simulink model "b6_pfc_rl"  (R2021b)
settings: Solver=FixedStepAuto  StartTime=0.0  StopTime=120.0  FixedStep=0.05  RelTol=1e-3
PreLoadFcn:
  | % Simulation parameters
  | %load exampleMap
  | 
  | % Lidar parameters
  | sensorOffset = [0,0];
  | scanAngles = linspace(-pi/2,pi/2,9)';
  | maxRange = 5;
InitFcn:
  | sampleTime = 0.05;
  | nMedianSize=3;
  | 
  | % Robot parameters
  | wheelRadius = 0.0335;
  | robotRadius = 0.116;
  | 
  | % Lidar parameters
  | sensorOffset = [0,0];
  | scanAngles = linspace(-pi/2,pi/2,9)';
  | maxRange = 5;
  | 
  | %%%%%%
  | ks=1;
  | c_ks=-1;
  | 
  | 
  | 
  | 
  | 
  | 
  | % Lidar parameters
  | sensorOffset = [0,0];
  | scanAngles = linspace(-pi/3,pi/3,20)';%y = linspace(x1,x2,n) 生成 n 个点。这些点的间距为 (x2-x1)/(n-1)。
  | maxRange = 0.4;
  | 
  | %%%%%%
  | ks=1;
  | 
  | 
  | 
  | 
  | 
  | A=0.3;
  | C=1.7;
  | B=(A+C)/2;
  | 
  | wp1=[A,A; B,A;  C,A; C,B;C,C; B,C; A,C;A,B];
  | bainjie2=[-0.5,-0.5;2.5,-0.5;-0.5,2.5;2.5,2.5;]
  | WAY_P=[wp1;wp1;wp1;wp1];
  | Target=[wp1;bainjie2];
  | 
  | %%%%%%%%%%%%%%%%%%%%%%%%%%%%%%%%%%%%%%%
  | Target_robot_4=[A  A]
  | Target_robot_5=[B  A]
  | Target_robot_6=[C  A]
  | 
  | Target_robot_1=[C  C]
  | Target_robot_2=[B  C]
  | Target_robot_3=[A  C]
  | 
  | 
  | %%%%%%%%%%%%%%%%%%%%%%%%%%%%%%%%%%%%
  | 
  | 
  | 
  | 
  | 
  | % paremeters of pure persuit
  | desired_v_robot_1=0.2
  | desired_w_robot_1=4
  | desired_lookahead_robot_1=0.2
  | 
  | % paremeters of recovery
  | recovery_w=0.5
  | 
  | 
  | 
  | 
  | 
  | %初始位置
  | x_1_0=1;
  | y_1_0=0;
  | yaw_1_0=0.0;
  | 
  | x_2_0=0.6;
  | y_2_0=0;
  | yaw_2_0=0;
  | 
  | x_3_0=0.3;
  | y_3_0=0;
  | yaw_3_0=0;
  | 
  | x_4_0=0;
  | y_4_0=0;
  | yaw_4_0=0;
  | 
  | x_5_0=-0.3;
  | y_5_0=0;
  | yaw_5_0=0;
  | 
  | x_6_0=-0.6;
  | y_6_0=0;
  | yaw_6_0=0;
  | 
  | init_pose_1=[x_1_0   y_1_0  yaw_1_0]';
  | init_pose_2=[x_2_0   y_2_0  yaw_2_0]';
  | init_pose_3=[x_3_0   y_3_0  yaw_3_0]';
  | init_pose_4=[x_4_0   y_4_0  yaw_4_0]';
  | 
  | init_pose_5=[x_5_0   y_5_0  yaw_5_0]';
  | init_pose_6=[x_6_0   y_6_0  yaw_6_0]';
undefined symbols (not defined in the file or in its folder): Angular, DiscIntNeverNeededParam, Linear, Pose, Twist
libraries: robotlib x42, dspstat3 x18, mobileRoboticsLib x13, robotmobilelib x6, simulink x2, robotalgslib x1
(part 1 of 3)
settings Model: Creator=scastro  LastModifiedBy=FCS
settings SolverCC: AlgebraicLoopSolver=TrustRegion
settings DataIOCC: ReturnWorkspaceOutputs=off
settings OptimizationCC: DefaultParameterBehavior=Inlined  EnhancedBackFolding=on  PassReuseOutputArgsAs=Individual arguments  ZeroExternalMemoryAtStartup=off  ZeroInternalMemoryAtStartup=off  InitFltsAndDblsToZero=on  MaxStackSize=64  OptimizeBlockOrder=speed  DifferentSizesBufferReuse=on  OptimizationCustomize=off  EfficientTunableParamExpr=on
settings DebuggingCC: ParameterTunabilityLossMsg=error  PregeneratedLibrarySubsystemCodeDiagnostic=none  SFMachineParentedDataDiag=warning  ArithmeticOperatorsInVariantConditions=warning
settings HardwareCC: ProdBitPerPointer=32  ProdBitPerSizeT=32  ProdBitPerPtrDiffT=32  ProdLargestAtomicFloat=None  ProdIntDivRoundTo=Undefined  ProdEndianess=Unspecified  ProdWordSize=32  ProdLongLongMode=on  ProdHWDeviceType=Generic->Unspecified (assume 32-bit Generic)  TargetLongLongMode=on
settings SFSimCC: SimUseLocalCustomCode=off  MATLABDynamicMemAlloc=off  CustomCodeUndefinedFunction=UseInterfaceOnly  SimTargetLang=C++
settings RTWCC: Description=Embedded Coder  SystemTargetFile=ert.tlc  HardwareBoard=Robot Operating System (ROS)  TLCOptions="-aInlineSetEventsForThisBaseRateFcn=TLC_FALSE -aSuppressMultiTaskScheduler=TLC_FALSE  -aRateBasedStepFcn=0"  TemplateMakefile=ert_default_tmf  RTWUseLocalCustomCode=off  Toolchain=Catkin  TargetLang=C++  GenerateGPUCode=CUDA
settings CodeAppCC: ForceParamTrailComments=on  IgnoreCustomStorageClasses=off  OperatorAnnotations=on  SimulinkDataObjDesc=on  SFDataObjDesc=on  InsertBlockDesc=on
settings ERTTargetCC: TargetLangStandard=C++11 (ISO)  CodeInterfacePackaging=C++ class  InlinedParameterPlacement=NonHierarchical  RootIOFormat=Structure reference  ERTCustomFileTemplate=example_file_process.tlc

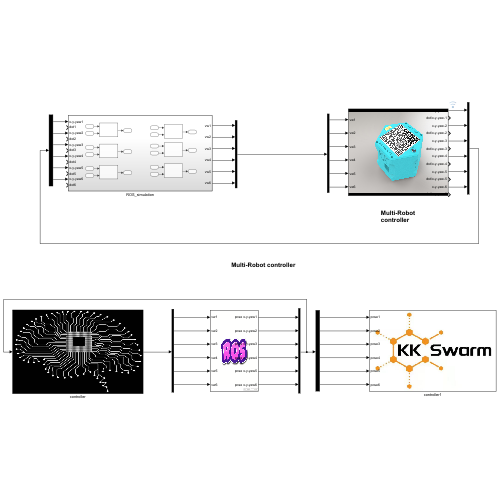
[thumbnail: Simulink's stored preview of the top-level diagram]
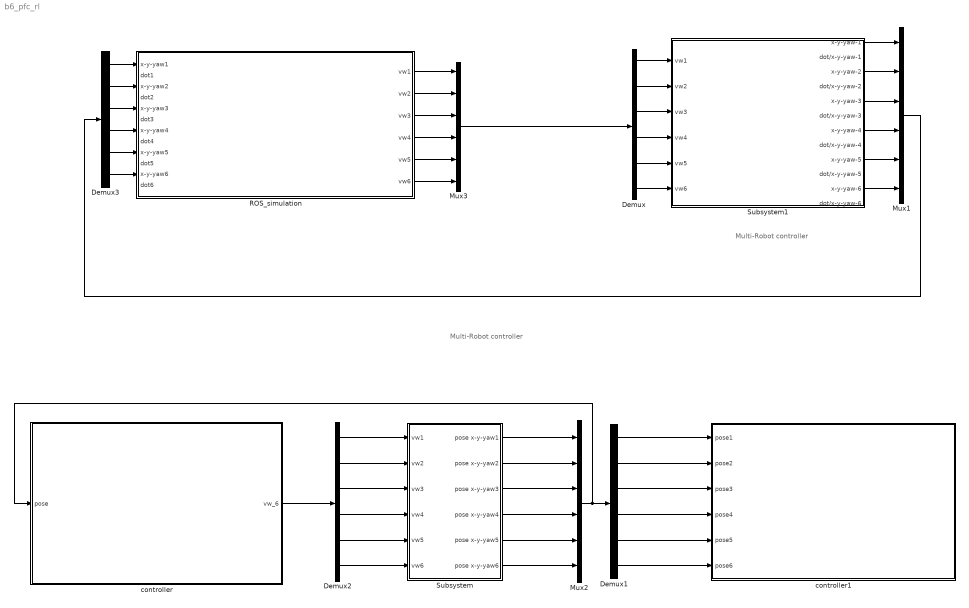
== system b6_pfc_rl ==
  note: Multi-Robot
      | controller
  note: Multi-Robot controller
  Demux{,1..3} (4 alike) : Demux  Outputs=6
  Mux1 : Mux  Inputs=6
  Mux2 : Mux  Inputs=6
  Mux3 : Mux  Inputs=6
  ROS_simulation : Subsystem
  Subsystem : Subsystem
      mask Display: image('$imagefile'); % 使用工具条上的 "编辑图像" 进行更改。
  Subsystem1 : Subsystem
      mask Display: image('$imagefile'); % 使用工具条上的 "编辑图像" 进行更改。
  controller : Subsystem
      mask Display: image('$imagefile'); % 使用工具条上的 "编辑图像" 进行更改。
  controller1 : Subsystem
      mask Display: image('$imagefile'); % 使用工具条上的 "编辑图像" 进行更改。
  wires:
  Demux/6 -> Subsystem1/6(vw6)
  ROS_simulation/3(vw3) -> Mux3/3
  Demux3/3 -> ROS_simulation/5(x-y-yaw3)
  Demux3/6 -> ROS_simulation/11(x-y-yaw6)
  Subsystem1/5(x-y-yaw-3) -> Mux1/3
  ROS_simulation/1(vw1) -> Mux3/1
  Mux3/1 -> Demux/1
  Demux/3 -> Subsystem1/3(vw3)
  Demux/4 -> Subsystem1/4(vw4)
  Demux3/4 -> ROS_simulation/7(x-y-yaw4)
  Mux1/1 -> Demux3/1
  Subsystem1/7(x-y-yaw-4) -> Mux1/4
  Demux3/2 -> ROS_simulation/3(x-y-yaw2)
  ROS_simulation/4(vw4) -> Mux3/4
  ROS_simulation/2(vw2) -> Mux3/2
  Demux/5 -> Subsystem1/5(vw5)
  Subsystem1/1(x-y-yaw-1) -> Mux1/1
  Demux/1 -> Subsystem1/1(vw1)
  ROS_simulation/6(vw6) -> Mux3/6
  ROS_simulation/5(vw5) -> Mux3/5
  Subsystem1/9(x-y-yaw-5) -> Mux1/5
  Demux/2 -> Subsystem1/2(vw2)
  Demux3/1 -> ROS_simulation/1(x-y-yaw1)
  Subsystem1/11(x-y-yaw-6) -> Mux1/6
  Demux3/5 -> ROS_simulation/9(x-y-yaw5)
  Subsystem1/3(x-y-yaw-2) -> Mux1/2
  Demux1/6 -> controller1/6(pose6)
  Subsystem/2(pose x-y-yaw2) -> Mux2/2
  Demux2/4 -> Subsystem/4(vw4)
  Demux1/5 -> controller1/5(pose5)
  Demux2/6 -> Subsystem/6(vw6)
  Mux2/1 -> controller/1(pose), Demux1/1
  Demux2/3 -> Subsystem/3(vw3)
  Demux1/4 -> controller1/4(pose4)
  Demux2/2 -> Subsystem/2(vw2)
  Demux2/5 -> Subsystem/5(vw5)
  Subsystem/4(pose x-y-yaw4) -> Mux2/4
  Demux1/3 -> controller1/3(pose3)
  Subsystem/6(pose x-y-yaw6) -> Mux2/6
  Demux1/1 -> controller1/1(pose1)
  Subsystem/1(pose x-y-yaw1) -> Mux2/1
  Subsystem/3(pose x-y-yaw3) -> Mux2/3
  Subsystem/5(pose x-y-yaw5) -> Mux2/5
  Demux1/2 -> controller1/2(pose2)
  Demux2/1 -> Subsystem/1(vw1)
  controller/1(vw_6) -> Demux2/1

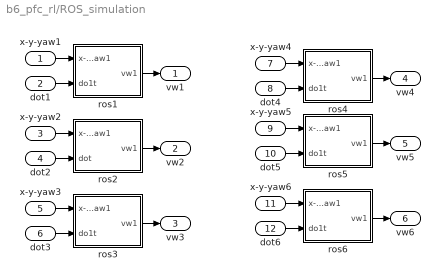
== system b6_pfc_rl/ROS_simulation ==
  x-y-yaw1 : Inport
  dot1 : Inport  Port=2
  x-y-yaw2 : Inport  Port=3
  dot2 : Inport  Port=4
  x-y-yaw3 : Inport  Port=5
  dot3 : Inport  Port=6
  x-y-yaw4 : Inport  Port=7
  dot4 : Inport  Port=8
  x-y-yaw5 : Inport  Port=9
  dot5 : Inport  Port=10
  x-y-yaw6 : Inport  Port=11
  dot6 : Inport  Port=12
  ros1 : Subsystem
  ros2 : Subsystem
  ros3 : Subsystem
  ros4 : Subsystem
  ros5 : Subsystem
  ros6 : Subsystem
  vw1 : Outport
  vw2 : Outport  Port=2
  vw3 : Outport  Port=3
  vw4 : Outport  Port=4
  vw5 : Outport  Port=5
  vw6 : Outport  Port=6
  wires:
  ros5/1(vw1) -> vw5/1
  ros2/1(vw1) -> vw2/1
  dot3/1 -> ros3/2(do1t)
  x-y-yaw5/1 -> ros5/1(x-y-yaw1)
  ros3/1(vw1) -> vw3/1
  dot2/1 -> ros2/2(dot)
  x-y-yaw2/1 -> ros2/1(x-y-yaw1)
  dot5/1 -> ros5/2(do1t)
  dot4/1 -> ros4/2(do1t)
  x-y-yaw4/1 -> ros4/1(x-y-yaw1)
  ros4/1(vw1) -> vw4/1
  x-y-yaw3/1 -> ros3/1(x-y-yaw1)
  dot6/1 -> ros6/2(do1t)
  x-y-yaw6/1 -> ros6/1(x-y-yaw1)
  dot1/1 -> ros1/2(do1t)
  ros6/1(vw1) -> vw6/1
  x-y-yaw1/1 -> ros1/1(x-y-yaw1)
  ros1/1(vw1) -> vw1/1

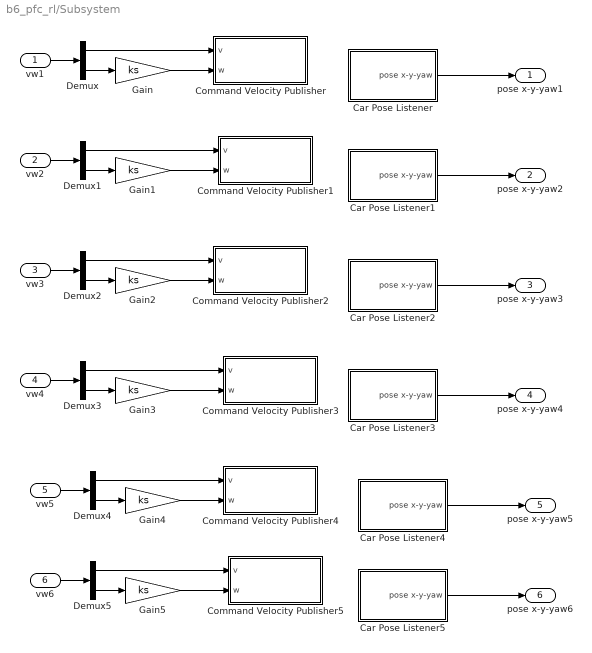
== system b6_pfc_rl/Subsystem ==
  vw1 : Inport
  vw2 : Inport  Port=2
  vw3 : Inport  Port=3
  vw4 : Inport  Port=4
  vw5 : Inport  Port=5
  vw6 : Inport  Port=6
  Car Pose Listener : Subsystem
  Car Pose Listener1 : Subsystem
  Car Pose Listener2 : Subsystem
  Car Pose Listener3 : Subsystem
  Car Pose Listener4 : Subsystem
  Car Pose Listener5 : Subsystem
  Command Velocity Publisher : Subsystem
  Command Velocity Publisher1 : Subsystem
  Command Velocity Publisher2 : Subsystem
  Command Velocity Publisher3 : Subsystem
  Command Velocity Publisher4 : Subsystem
  Command Velocity Publisher5 : Subsystem
  Demux{,1..5} (6 alike) : Demux  Outputs=2
  Gain{,1..5} (6 alike) : Gain  Gain=ks
  pose x-y-yaw1 : Outport
  pose x-y-yaw2 : Outport  Port=2
  pose x-y-yaw3 : Outport  Port=3
  pose x-y-yaw4 : Outport  Port=4
  pose x-y-yaw5 : Outport  Port=5
  pose x-y-yaw6 : Outport  Port=6
  wires:
  Gain/1 -> Command Velocity Publisher/2(w)
  Demux/2 -> Gain/1
  Car Pose Listener/1(pose x-y-yaw) -> pose x-y-yaw1/1
  Demux/1 -> Command Velocity Publisher/1(v)
  vw1/1 -> Demux/1
  Car Pose Listener1/1(pose x-y-yaw) -> pose x-y-yaw2/1
  Gain1/1 -> Command Velocity Publisher1/2(w)
  vw2/1 -> Demux1/1
  Demux1/2 -> Gain1/1
  Demux1/1 -> Command Velocity Publisher1/1(v)
  Car Pose Listener2/1(pose x-y-yaw) -> pose x-y-yaw3/1
  Gain2/1 -> Command Velocity Publisher2/2(w)
  vw3/1 -> Demux2/1
  Demux2/2 -> Gain2/1
  Demux2/1 -> Command Velocity Publisher2/1(v)
  Car Pose Listener3/1(pose x-y-yaw) -> pose x-y-yaw4/1
  Gain3/1 -> Command Velocity Publisher3/2(w)
  vw4/1 -> Demux3/1
  Demux3/2 -> Gain3/1
  Demux3/1 -> Command Velocity Publisher3/1(v)
  Car Pose Listener4/1(pose x-y-yaw) -> pose x-y-yaw5/1
  Gain4/1 -> Command Velocity Publisher4/2(w)
  vw5/1 -> Demux4/1
  Demux4/2 -> Gain4/1
  Car Pose Listener5/1(pose x-y-yaw) -> pose x-y-yaw6/1
  Gain5/1 -> Command Velocity Publisher5/2(w)
  vw6/1 -> Demux5/1
  Demux5/2 -> Gain5/1
  Demux5/1 -> Command Velocity Publisher5/1(v)
  Demux4/1 -> Command Velocity Publisher4/1(v)

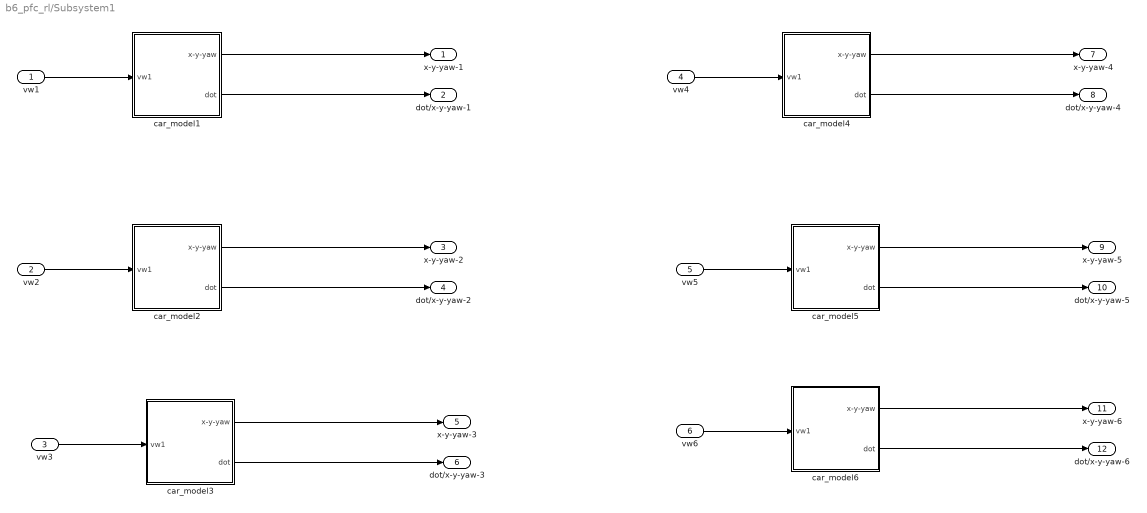
== system b6_pfc_rl/Subsystem1 ==
  vw1 : Inport
  vw2 : Inport  Port=2
  vw3 : Inport  Port=3
  vw4 : Inport  Port=4
  vw5 : Inport  Port=5
  vw6 : Inport  Port=6
  car_model1 : Subsystem
  car_model2 : Subsystem
  car_model3 : Subsystem
  car_model4 : Subsystem
  car_model5 : Subsystem
  car_model6 : Subsystem
  x-y-yaw-1 : Outport
  dot/x-y-yaw-1 : Outport  Port=2
  x-y-yaw-2 : Outport  Port=3
  dot/x-y-yaw-2 : Outport  Port=4
  x-y-yaw-3 : Outport  Port=5
  dot/x-y-yaw-3 : Outport  Port=6
  x-y-yaw-4 : Outport  Port=7
  dot/x-y-yaw-4 : Outport  Port=8
  x-y-yaw-5 : Outport  Port=9
  dot/x-y-yaw-5 : Outport  Port=10
  x-y-yaw-6 : Outport  Port=11
  dot/x-y-yaw-6 : Outport  Port=12
  wires:
  car_model1/1(x-y-yaw) -> x-y-yaw-1/1
  vw1/1 -> car_model1/1(vw1)
  car_model1/2(dot) -> dot/x-y-yaw-1/1
  car_model2/2(dot) -> dot/x-y-yaw-2/1
  vw2/1 -> car_model2/1(vw1)
  car_model2/1(x-y-yaw) -> x-y-yaw-2/1
  car_model3/1(x-y-yaw) -> x-y-yaw-3/1
  vw3/1 -> car_model3/1(vw1)
  car_model3/2(dot) -> dot/x-y-yaw-3/1
  car_model4/1(x-y-yaw) -> x-y-yaw-4/1
  vw4/1 -> car_model4/1(vw1)
  car_model4/2(dot) -> dot/x-y-yaw-4/1
  car_model5/1(x-y-yaw) -> x-y-yaw-5/1
  vw5/1 -> car_model5/1(vw1)
  car_model5/2(dot) -> dot/x-y-yaw-5/1
  car_model6/1(x-y-yaw) -> x-y-yaw-6/1
  vw6/1 -> car_model6/1(vw1)
  car_model6/2(dot) -> dot/x-y-yaw-6/1

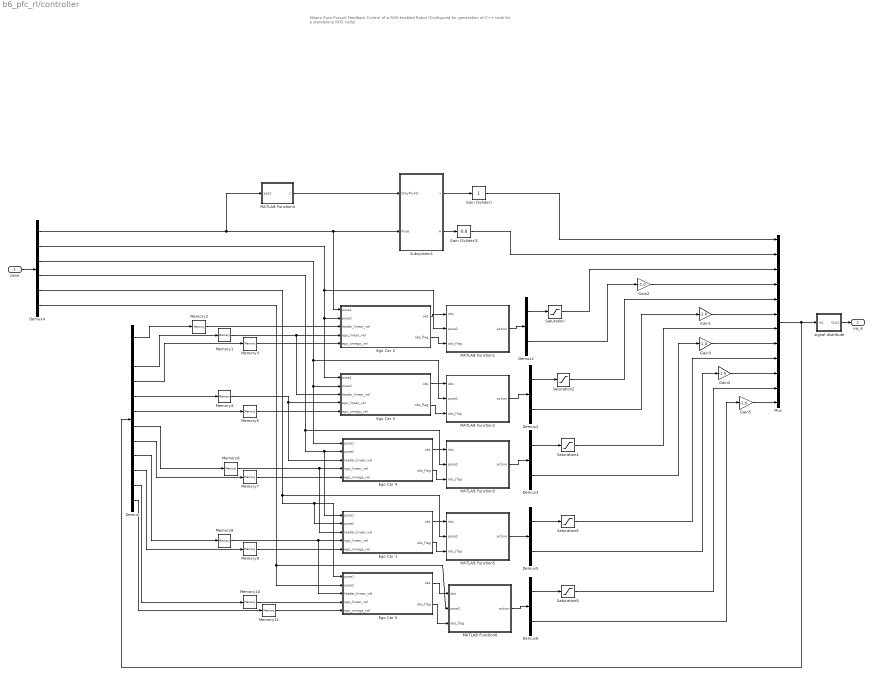
== system b6_pfc_rl/controller ==
  note: Misaro Pure Pursuit Feedback Control of a ROS-enabled Robot
      | (Configured for generation of C++ code for a standalone ROS node)
  pose : Inport
  Demux : Demux  Outputs=12
  Demux{1..3,5..6} (5 alike) : Demux  Outputs=2
  Demux4 : Demux  Outputs=6
  Ego Car 1 : Subsystem
  Ego Car 2 : Subsystem
  Ego Car 3 : Subsystem
  Ego Car 4 : Subsystem
  Ego Car 5 : Subsystem
  Gain (Svlider) : simulink/Math Operations/Slider Gain  gain=1  low=0.1  high=10
  Gain (Svlider)1 : simulink/Math Operations/Slider Gain  gain=0.8  low=0.1  high=3
  Gain{1..5} (5 alike) : Gain  Gain=-1.0
  MATLAB Function1 : MATLAB Function  TreatAsAtomicUnit=on
  MATLAB Function2 : MATLAB Function  TreatAsAtomicUnit=on
  MATLAB Function3 : MATLAB Function  TreatAsAtomicUnit=on
  MATLAB Function4 : MATLAB Function  TreatAsAtomicUnit=on
  MATLAB Function5 : MATLAB Function  TreatAsAtomicUnit=on
  MATLAB Function6 : MATLAB Function  TreatAsAtomicUnit=on
  Memory{1..2,4,6,8,10} (6 alike) : Memory  InitialCondition=0.2
  Memory{3,5,7,9,11} (5 alike) : Memory
  Mux : Mux  Inputs=12
  Saturation{,2,4,6,8} (5 alike) : Saturate  LowerLimit=0.1  OutDataTypeStr=double
  Subsystem1 : Subsystem
  signal distribute : Subsystem
  vw_6 : Outport
  wires:
  Demux4/1 -> MATLAB Function4/1(pos1), Ego Car 2/1(pose1), Subsystem1/2(Pose)
  Demux/1 -> Memory2/1
  Demux/3 -> Memory1/1
  Demux/4 -> Memory3/1
  Demux/5 -> Memory4/1
  Demux/6 -> Memory5/1
  Demux/7 -> Memory6/1
  Demux/8 -> Memory7/1
  Demux4/2 -> MATLAB Function1/2(pose2), Ego Car 3/1(pose1), Ego Car 2/2(pose2)
  Demux4/3 -> MATLAB Function2/2(pose2), Ego Car 4/1(pose1), Ego Car 3/2(pose2)
  Demux4/4 -> MATLAB Function3/2(pose2), Ego Car 1/1(pose1), Ego Car 4/2(pose2)
  Subsystem1/1(v) -> Gain (Svlider)/1
  Memory2/1 -> Ego Car 2/3(leader_linear_vel)
  Memory1/1 -> Ego Car 3/3(leader_linear_vel), Ego Car 2/4(ego_linear_vel)
  Memory3/1 -> Ego Car 2/5(ego_omega_vel)
  Demux1/1 -> Saturation/1
  Saturation/1 -> Mux/3
  Subsystem1/2(w) -> Gain (Svlider)1/1
  Demux1/2 -> Gain2/1
  Memory4/1 -> Ego Car 4/3(leader_linear_vel), Ego Car 3/4(ego_linear_vel)
  Memory5/1 -> Ego Car 3/5(ego_omega_vel)
  Demux2/1 -> Saturation2/1
  Saturation2/1 -> Mux/5
  Demux2/2 -> Gain1/1
  Gain1/1 -> Mux/6
  Memory6/1 -> Ego Car 1/3(leader_linear_vel), Ego Car 4/4(ego_linear_vel)
  Memory7/1 -> Ego Car 4/5(ego_omega_vel)
  Demux3/1 -> Saturation4/1
  Saturation4/1 -> Mux/7
  Demux3/2 -> Gain3/1
  Gain3/1 -> Mux/8
  pose/1 -> Demux4/1
  Mux/1 -> Demux/1, signal distribute/1(In1)
  signal distribute/1(Out1) -> vw_6/1
  MATLAB Function4/1(z) -> Subsystem1/1(WayPoints)
  Gain (Svlider)/1 -> Mux/1
  Gain2/1 -> Mux/4
  Gain (Svlider)1/1 -> Mux/2
  Ego Car 3/1(obs) -> MATLAB Function2/1(obs)
  Ego Car 3/2(obs_flag) -> MATLAB Function2/3(obs_flag)
  MATLAB Function2/1(action) -> Demux2/1
  Ego Car 4/2(obs_flag) -> MATLAB Function3/3(obs_flag)
  Ego Car 4/1(obs) -> MATLAB Function3/1(obs)
  MATLAB Function3/1(action) -> Demux3/1
  MATLAB Function1/1(action) -> Demux1/1
  Ego Car 2/2(obs_flag) -> MATLAB Function1/3(obs_flag)
  Ego Car 2/1(obs) -> MATLAB Function1/1(obs)
  Demux/9 -> Memory8/1
  Demux/10 -> Memory9/1
  Memory8/1 -> Ego Car 5/3(leader_linear_vel), Ego Car 1/4(ego_linear_vel)
  Memory9/1 -> Ego Car 1/5(ego_omega_vel)
  Demux4/5 -> MATLAB Function5/2(pose2), Ego Car 5/1(pose1), Ego Car 1/2(pose2)
  Ego Car 1/1(obs) -> MATLAB Function5/1(obs)
  Ego Car 1/2(obs_flag) -> MATLAB Function5/3(obs_flag)
  Demux5/1 -> Saturation6/1
  MATLAB Function5/1(action) -> Demux5/1
  Saturation6/1 -> Mux/9
  Gain4/1 -> Mux/10
  Demux5/2 -> Gain4/1
  Demux/11 -> Memory10/1
  Memory10/1 -> Ego Car 5/4(ego_linear_vel)
  Demux/12 -> Memory11/1
  Memory11/1 -> Ego Car 5/5(ego_omega_vel)
  Demux4/6 -> MATLAB Function6/2(pose2), Ego Car 5/2(pose2)
  Ego Car 5/1(obs) -> MATLAB Function6/1(obs)
  Ego Car 5/2(obs_flag) -> MATLAB Function6/3(obs_flag)
  Demux6/1 -> Saturation8/1
  MATLAB Function6/1(action) -> Demux6/1
  Saturation8/1 -> Mux/11
  Gain5/1 -> Mux/12
  Demux6/2 -> Gain5/1

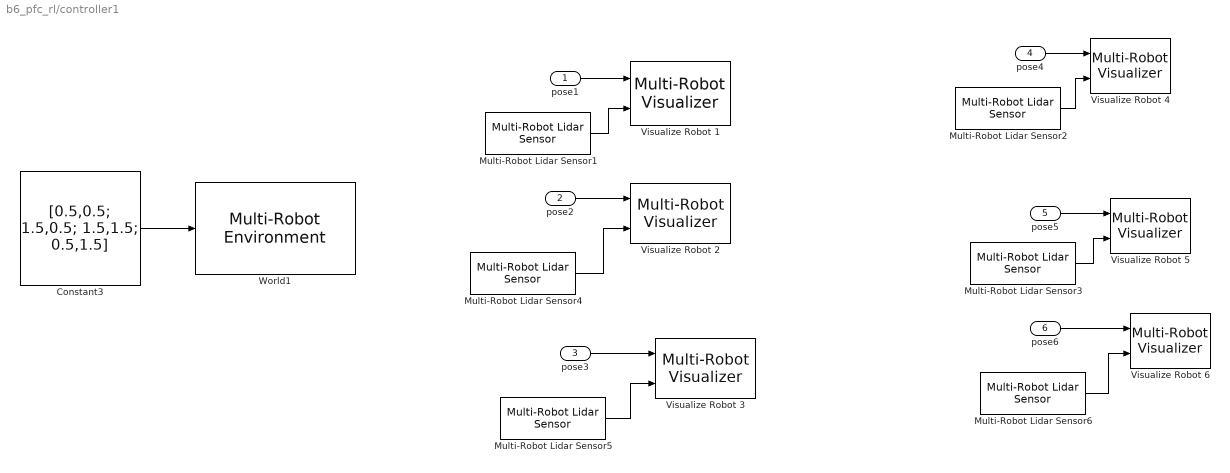
== system b6_pfc_rl/controller1 ==
  pose1 : Inport
  pose2 : Inport  Port=2
  pose3 : Inport  Port=3
  pose4 : Inport  Port=4
  pose5 : Inport  Port=5
  pose6 : Inport  Port=6
  Constant3 : Constant  Value="[0.5,0.5; 1.5,0.5;  1.5,1.5;  0.5,1.5]"
  Multi-Robot Lidar Sensor1 : mobileRoboticsLib/Environments/Multi-Robot Lidar Sensor  robotIdx=1  sensorOffset=sensorOffset  scanAngles=scanAngles  maxRange=maxRange
      settings: SourceProductName=Mobile Robotics Simulation Toolbox
  Multi-Robot Lidar Sensor2 : mobileRoboticsLib/Environments/Multi-Robot Lidar Sensor  robotIdx=4  sensorOffset=sensorOffset  scanAngles=scanAngles  maxRange=maxRange
      settings: SourceProductName=Mobile Robotics Simulation Toolbox
  Multi-Robot Lidar Sensor3 : mobileRoboticsLib/Environments/Multi-Robot Lidar Sensor  robotIdx=5  sensorOffset=sensorOffset  scanAngles=scanAngles  maxRange=maxRange
      settings: SourceProductName=Mobile Robotics Simulation Toolbox
  Multi-Robot Lidar Sensor4 : mobileRoboticsLib/Environments/Multi-Robot Lidar Sensor  robotIdx=2  sensorOffset=sensorOffset  scanAngles=scanAngles  maxRange=maxRange
      settings: SourceProductName=Mobile Robotics Simulation Toolbox
  Multi-Robot Lidar Sensor5 : mobileRoboticsLib/Environments/Multi-Robot Lidar Sensor  robotIdx=3  sensorOffset=sensorOffset  scanAngles=scanAngles  maxRange=maxRange
      settings: SourceProductName=Mobile Robotics Simulation Toolbox
  Multi-Robot Lidar Sensor6 : mobileRoboticsLib/Environments/Multi-Robot Lidar Sensor  robotIdx=6  sensorOffset=sensorOffset  scanAngles=scanAngles  maxRange=maxRange
      settings: SourceProductName=Mobile Robotics Simulation Toolbox
  Visualize Robot 1 : mobileRoboticsLib/Environments/Multi-Robot Visualizer  idx=1  radius=robotRadius  robotColor=[0 0 1]  showTraj=off  hasLidar=on  sensorOffset=sensorOffset  scanAngles=scanAngles  maxNumScans=0  hasObjDetector=off  objDetectorOffset=[0,0]  objDetectorAngle=0  objDetectorFOV=pi/2  objDetectorMaxRange=5  hasRobotDetector=off  robotDetectorOffset=[0,0]  robotDetectorAngle=0  robotDetectorFOV=pi/3  robotDetectorMaxRange=5  robotDetectorNumDetections=0
      settings: SourceProductName=Mobile Robotics Simulation Toolbox
  Visualize Robot 2 : mobileRoboticsLib/Environments/Multi-Robot Visualizer  idx=2  radius=robotRadius  robotColor=[0 1 0]  showTraj=on  hasLidar=on  sensorOffset=sensorOffset  scanAngles=scanAngles  maxNumScans=0  hasObjDetector=off  objDetectorOffset=[0,0]  objDetectorAngle=0  objDetectorFOV=pi/2  objDetectorMaxRange=5  hasRobotDetector=off  robotDetectorOffset=[0,0]  robotDetectorAngle=0  robotDetectorFOV=pi/3  robotDetectorMaxRange=5  robotDetectorNumDetections=0
      settings: SourceProductName=Mobile Robotics Simulation Toolbox
  Visualize Robot 3 : mobileRoboticsLib/Environments/Multi-Robot Visualizer  idx=3  radius=robotRadius  robotColor=[0 1 0]  showTraj=off  hasLidar=on  sensorOffset=sensorOffset  scanAngles=scanAngles  maxNumScans=0  hasObjDetector=off  objDetectorOffset=[0,0]  objDetectorAngle=0  objDetectorFOV=pi/2  objDetectorMaxRange=5  hasRobotDetector=off  robotDetectorOffset=[0,0]  robotDetectorAngle=0  robotDetectorFOV=pi/3  robotDetectorMaxRange=5  robotDetectorNumDetections=0
      settings: SourceProductName=Mobile Robotics Simulation Toolbox
  Visualize Robot 4 : mobileRoboticsLib/Environments/Multi-Robot Visualizer  idx=4  radius=robotRadius  robotColor=[1 0 0]  showTraj=on  hasLidar=on  sensorOffset=sensorOffset  scanAngles=scanAngles  maxNumScans=0  hasObjDetector=off  objDetectorOffset=[0,0]  objDetectorAngle=0  objDetectorFOV=pi/2  objDetectorMaxRange=5  hasRobotDetector=off  robotDetectorOffset=[0,0]  robotDetectorAngle=0  robotDetectorFOV=pi/3  robotDetectorMaxRange=5  robotDetectorNumDetections=0
      settings: SourceProductName=Mobile Robotics Simulation Toolbox
  Visualize Robot 5 : mobileRoboticsLib/Environments/Multi-Robot Visualizer  idx=5  radius=robotRadius  robotColor=[1 0 1]  showTraj=off  hasLidar=on  sensorOffset=sensorOffset  scanAngles=scanAngles  maxNumScans=0  hasObjDetector=off  objDetectorOffset=[0,0]  objDetectorAngle=0  objDetectorFOV=pi/2  objDetectorMaxRange=5  hasRobotDetector=off  robotDetectorOffset=[0,0]  robotDetectorAngle=0  robotDetectorFOV=pi/3  robotDetectorMaxRange=5  robotDetectorNumDetections=0
      settings: SourceProductName=Mobile Robotics Simulation Toolbox
  Visualize Robot 6 : mobileRoboticsLib/Environments/Multi-Robot Visualizer  idx=6  radius=robotRadius  robotColor=[1 0 0]  showTraj=off  hasLidar=on  sensorOffset=sensorOffset  scanAngles=scanAngles  maxNumScans=0  hasObjDetector=off  objDetectorOffset=[0,0]  objDetectorAngle=0  objDetectorFOV=pi/2  objDetectorMaxRange=5  hasRobotDetector=off  robotDetectorOffset=[0,0]  robotDetectorAngle=0  robotDetectorFOV=pi/3  robotDetectorMaxRange=5  robotDetectorNumDetections=0
      settings: SourceProductName=Mobile Robotics Simulation Toolbox
  World1 : mobileRoboticsLib/Environments/Multi-Robot Environment  numRobots=6  showWaypoints=on  showObjects=off  objectColors=[1 0 0;0 1 0;0 0 1]  objectMarkers='s'  showRobotIds=on  plotSensorLines=on
      settings: SourceProductName=Mobile Robotics Simulation Toolbox
  wires:
  Multi-Robot Lidar Sensor5/1 -> Visualize Robot 3/2
  Multi-Robot Lidar Sensor4/1 -> Visualize Robot 2/2
  pose2/1 -> Visualize Robot 2/1
  Multi-Robot Lidar Sensor1/1 -> Visualize Robot 1/2
  Multi-Robot Lidar Sensor6/1 -> Visualize Robot 6/2
  Multi-Robot Lidar Sensor2/1 -> Visualize Robot 4/2
  pose6/1 -> Visualize Robot 6/1
  pose1/1 -> Visualize Robot 1/1
  pose4/1 -> Visualize Robot 4/1
  pose5/1 -> Visualize Robot 5/1
  Multi-Robot Lidar Sensor3/1 -> Visualize Robot 5/2
  pose3/1 -> Visualize Robot 3/1
  Constant3/1 -> World1/1

== system b6_pfc_rl/ROS_simulation/ros1 ==
  x-y-yaw1 : Inport
  do1t : Inport  Port=2
  " [x y theta]" : Demux  Outputs=3
  " [x y theta]1" : Demux  Outputs=3
  Blank Message : robotlib/Blank Message  messageClass=Message  entityType=nav_msgs/Odometry  messageType=nav_msgs/Odometry  SampleTime=inf  legacyBusStruct=off
  Bus Assignment1 : BusAssignment  DialogController=Simulink.DDGSource_BusAssignment  AssignedSignals=Pose.Pose.Position.X,Pose.Pose.Position.Y,Pose.Pose.Orientation.Z,Pose.Pose.Orientation.W,Twist.Twist.Linear.X,Twist.Twist.Linear.Y,Twist.Twist.Angular.Z
  MATLAB Function : MATLAB Function  TreatAsAtomicUnit=on
  MATLAB Function3 : MATLAB Function  TreatAsAtomicUnit=on
  Mux6 : Mux  Inputs=2
  Publish2 : robotlib/Publish  topicSource=Specify your own  topic=/robot_1/pose  messageType=nav_msgs/Odometry  legacyBusStruct=off  messageQueueLength=105
  Subscribe1 : robotlib/Subscribe  topicSource=Specify your own  topic=/robot_1/cmd_vel  messageType=geometry_msgs/Twist  SampleTime=-1  legacyBusStruct=off  messageQueueLength=51
  Terminator : Terminator
  Terminator1 : Terminator
  Zero-Order Hold : ZeroOrderHold  SampleTime=0.1
  Zero-Order Hold1 : ZeroOrderHold  SampleTime=0.1
  vw1 : Outport
  wires:
  " [x y theta]"/1 -> Bus Assignment1/2
  Blank Message/1 -> Bus Assignment1/1
  x-y-yaw1/1 -> Zero-Order Hold/1
  " [x y theta]"/2 -> Bus Assignment1/3
  " [x y theta]1"/2 -> Bus Assignment1/7
  " [x y theta]"/3 -> MATLAB Function/1(yaw)
  " [x y theta]1"/3 -> Bus Assignment1/8
  MATLAB Function/4(w) -> Bus Assignment1/5
  MATLAB Function/3(z) -> Bus Assignment1/4
  " [x y theta]1"/1 -> Bus Assignment1/6
  Bus Assignment1/1 -> Publish2/1
  do1t/1 -> Zero-Order Hold1/1
  MATLAB Function/1(x) -> Terminator/1
  MATLAB Function/2(y) -> Terminator1/1
  Zero-Order Hold/1 -> " [x y theta]"/1
  Zero-Order Hold1/1 -> " [x y theta]1"/1
  Mux6/1 -> vw1/1
  MATLAB Function3/2(wref) -> Mux6/2
  MATLAB Function3/1(vref) -> Mux6/1
  Subscribe1/1 -> MATLAB Function3/1(IsNew)
  Subscribe1/2 -> MATLAB Function3/2(cmdMsg)

== system b6_pfc_rl/ROS_simulation/ros2 ==
  x-y-yaw1 : Inport
  dot : Inport  Port=2
  " [x y theta]" : Demux  Outputs=3
  " [x y theta]1" : Demux  Outputs=3
  Blank Message : robotlib/Blank Message  messageClass=Message  entityType=nav_msgs/Odometry  messageType=nav_msgs/Odometry  SampleTime=inf  legacyBusStruct=off
  Bus Assignment1 : BusAssignment  DialogController=Simulink.DDGSource_BusAssignment  AssignedSignals=Pose.Pose.Position.X,Pose.Pose.Position.Y,Pose.Pose.Orientation.Z,Pose.Pose.Orientation.W,Twist.Twist.Linear.X,Twist.Twist.Linear.Y,Twist.Twist.Angular.Z
  MATLAB Function : MATLAB Function  TreatAsAtomicUnit=on
  MATLAB Function3 : MATLAB Function  TreatAsAtomicUnit=on
  Mux6 : Mux  Inputs=2
  Publish2 : robotlib/Publish  topicSource=Specify your own  topic=/robot_2/pose  messageType=nav_msgs/Odometry  legacyBusStruct=off  messageQueueLength=105
  Subscribe1 : robotlib/Subscribe  topicSource=Specify your own  topic=/robot_2/cmd_vel  messageType=geometry_msgs/Twist  SampleTime=-1  legacyBusStruct=off  messageQueueLength=51
  Terminator : Terminator
  Terminator1 : Terminator
  Zero-Order Hold : ZeroOrderHold  SampleTime=0.1
  Zero-Order Hold1 : ZeroOrderHold  SampleTime=0.1
  vw1 : Outport
  wires:
  " [x y theta]"/1 -> Bus Assignment1/2
  Blank Message/1 -> Bus Assignment1/1
  x-y-yaw1/1 -> Zero-Order Hold/1
  " [x y theta]"/2 -> Bus Assignment1/3
  " [x y theta]1"/2 -> Bus Assignment1/7
  " [x y theta]"/3 -> MATLAB Function/1(yaw)
  " [x y theta]1"/3 -> Bus Assignment1/8
  MATLAB Function/4(w) -> Bus Assignment1/5
  MATLAB Function/3(z) -> Bus Assignment1/4
  " [x y theta]1"/1 -> Bus Assignment1/6
  Bus Assignment1/1 -> Publish2/1
  dot/1 -> Zero-Order Hold1/1
  MATLAB Function/1(x) -> Terminator/1
  MATLAB Function/2(y) -> Terminator1/1
  Zero-Order Hold/1 -> " [x y theta]"/1
  Zero-Order Hold1/1 -> " [x y theta]1"/1
  MATLAB Function3/1(vref) -> Mux6/1
  MATLAB Function3/2(wref) -> Mux6/2
  Subscribe1/1 -> MATLAB Function3/1(IsNew)
  Subscribe1/2 -> MATLAB Function3/2(cmdMsg)
  Mux6/1 -> vw1/1

== system b6_pfc_rl/ROS_simulation/ros3 ==
  x-y-yaw1 : Inport
  do1t : Inport  Port=2
  " [x y theta]" : Demux  Outputs=3
  " [x y theta]1" : Demux  Outputs=3
  Blank Message : robotlib/Blank Message  messageClass=Message  entityType=nav_msgs/Odometry  messageType=nav_msgs/Odometry  SampleTime=inf  legacyBusStruct=off
  Bus Assignment1 : BusAssignment  DialogController=Simulink.DDGSource_BusAssignment  AssignedSignals=Pose.Pose.Position.X,Pose.Pose.Position.Y,Pose.Pose.Orientation.Z,Pose.Pose.Orientation.W,Twist.Twist.Linear.X,Twist.Twist.Linear.Y,Twist.Twist.Angular.Z
  MATLAB Function : MATLAB Function  TreatAsAtomicUnit=on
  MATLAB Function3 : MATLAB Function  TreatAsAtomicUnit=on
  Mux6 : Mux  Inputs=2
  Publish2 : robotlib/Publish  topicSource=Specify your own  topic=/robot_3/pose  messageType=nav_msgs/Odometry  legacyBusStruct=off  messageQueueLength=105
  Subscribe1 : robotlib/Subscribe  topicSource=Specify your own  topic=/robot_3/cmd_vel  messageType=geometry_msgs/Twist  SampleTime=-1  legacyBusStruct=off  messageQueueLength=51
  Terminator : Terminator
  Terminator1 : Terminator
  Zero-Order Hold : ZeroOrderHold  SampleTime=0.1
  Zero-Order Hold1 : ZeroOrderHold  SampleTime=0.1
  vw1 : Outport
  wires:
  " [x y theta]"/1 -> Bus Assignment1/2
  Blank Message/1 -> Bus Assignment1/1
  x-y-yaw1/1 -> Zero-Order Hold/1
  " [x y theta]"/2 -> Bus Assignment1/3
  " [x y theta]1"/2 -> Bus Assignment1/7
  " [x y theta]"/3 -> MATLAB Function/1(yaw)
  " [x y theta]1"/3 -> Bus Assignment1/8
  MATLAB Function/4(w) -> Bus Assignment1/5
  MATLAB Function/3(z) -> Bus Assignment1/4
  " [x y theta]1"/1 -> Bus Assignment1/6
  Bus Assignment1/1 -> Publish2/1
  do1t/1 -> Zero-Order Hold1/1
  MATLAB Function/1(x) -> Terminator/1
  MATLAB Function/2(y) -> Terminator1/1
  Zero-Order Hold/1 -> " [x y theta]"/1
  Zero-Order Hold1/1 -> " [x y theta]1"/1
  MATLAB Function3/1(vref) -> Mux6/1
  MATLAB Function3/2(wref) -> Mux6/2
  Subscribe1/1 -> MATLAB Function3/1(IsNew)
  Subscribe1/2 -> MATLAB Function3/2(cmdMsg)
  Mux6/1 -> vw1/1

== system b6_pfc_rl/ROS_simulation/ros4 ==
  x-y-yaw1 : Inport
  do1t : Inport  Port=2
  " [x y theta]" : Demux  Outputs=3
  " [x y theta]1" : Demux  Outputs=3
  Blank Message : robotlib/Blank Message  messageClass=Message  entityType=nav_msgs/Odometry  messageType=nav_msgs/Odometry  SampleTime=inf  legacyBusStruct=off
  Bus Assignment1 : BusAssignment  DialogController=Simulink.DDGSource_BusAssignment  AssignedSignals=Pose.Pose.Position.X,Pose.Pose.Position.Y,Pose.Pose.Orientation.Z,Pose.Pose.Orientation.W,Twist.Twist.Linear.X,Twist.Twist.Linear.Y,Twist.Twist.Angular.Z
  MATLAB Function : MATLAB Function  TreatAsAtomicUnit=on
  MATLAB Function3 : MATLAB Function  TreatAsAtomicUnit=on
  Mux6 : Mux  Inputs=2
  Publish2 : robotlib/Publish  topicSource=Specify your own  topic=/robot_4/pose  messageType=nav_msgs/Odometry  legacyBusStruct=off  messageQueueLength=105
  Subscribe1 : robotlib/Subscribe  topicSource=Specify your own  topic=/robot_4/cmd_vel  messageType=geometry_msgs/Twist  SampleTime=-1  legacyBusStruct=off  messageQueueLength=51
  Terminator : Terminator
  Terminator1 : Terminator
  Zero-Order Hold : ZeroOrderHold  SampleTime=0.1
  Zero-Order Hold1 : ZeroOrderHold  SampleTime=0.1
  vw1 : Outport
  wires:
  " [x y theta]"/1 -> Bus Assignment1/2
  Blank Message/1 -> Bus Assignment1/1
  x-y-yaw1/1 -> Zero-Order Hold/1
  " [x y theta]"/2 -> Bus Assignment1/3
  " [x y theta]1"/2 -> Bus Assignment1/7
  " [x y theta]"/3 -> MATLAB Function/1(yaw)
  " [x y theta]1"/3 -> Bus Assignment1/8
  MATLAB Function/4(w) -> Bus Assignment1/5
  MATLAB Function/3(z) -> Bus Assignment1/4
  " [x y theta]1"/1 -> Bus Assignment1/6
  Bus Assignment1/1 -> Publish2/1
  do1t/1 -> Zero-Order Hold1/1
  MATLAB Function/1(x) -> Terminator/1
  MATLAB Function/2(y) -> Terminator1/1
  Zero-Order Hold/1 -> " [x y theta]"/1
  Zero-Order Hold1/1 -> " [x y theta]1"/1
  MATLAB Function3/1(vref) -> Mux6/1
  MATLAB Function3/2(wref) -> Mux6/2
  Subscribe1/1 -> MATLAB Function3/1(IsNew)
  Subscribe1/2 -> MATLAB Function3/2(cmdMsg)
  Mux6/1 -> vw1/1

== system b6_pfc_rl/ROS_simulation/ros5 ==
  x-y-yaw1 : Inport
  do1t : Inport  Port=2
  " [x y theta]" : Demux  Outputs=3
  " [x y theta]1" : Demux  Outputs=3
  Blank Message : robotlib/Blank Message  messageClass=Message  entityType=nav_msgs/Odometry  messageType=nav_msgs/Odometry  SampleTime=inf  legacyBusStruct=off
  Bus Assignment1 : BusAssignment  DialogController=Simulink.DDGSource_BusAssignment  AssignedSignals=Pose.Pose.Position.X,Pose.Pose.Position.Y,Pose.Pose.Orientation.Z,Pose.Pose.Orientation.W,Twist.Twist.Linear.X,Twist.Twist.Linear.Y,Twist.Twist.Angular.Z
  MATLAB Function : MATLAB Function  TreatAsAtomicUnit=on
  MATLAB Function3 : MATLAB Function  TreatAsAtomicUnit=on
  Mux6 : Mux  Inputs=2
  Publish2 : robotlib/Publish  topicSource=Specify your own  topic=/robot_5/pose  messageType=nav_msgs/Odometry  legacyBusStruct=off  messageQueueLength=105
  Subscribe1 : robotlib/Subscribe  topicSource=Specify your own  topic=/robot_5/cmd_vel  messageType=geometry_msgs/Twist  SampleTime=-1  legacyBusStruct=off  messageQueueLength=51
  Terminator : Terminator
  Terminator1 : Terminator
  Zero-Order Hold : ZeroOrderHold  SampleTime=0.1
  Zero-Order Hold1 : ZeroOrderHold  SampleTime=0.1
  vw1 : Outport
  wires:
  " [x y theta]"/1 -> Bus Assignment1/2
  Blank Message/1 -> Bus Assignment1/1
  x-y-yaw1/1 -> Zero-Order Hold/1
  " [x y theta]"/2 -> Bus Assignment1/3
  " [x y theta]1"/2 -> Bus Assignment1/7
  " [x y theta]"/3 -> MATLAB Function/1(yaw)
  " [x y theta]1"/3 -> Bus Assignment1/8
  MATLAB Function/4(w) -> Bus Assignment1/5
  MATLAB Function/3(z) -> Bus Assignment1/4
  " [x y theta]1"/1 -> Bus Assignment1/6
  Bus Assignment1/1 -> Publish2/1
  do1t/1 -> Zero-Order Hold1/1
  MATLAB Function/1(x) -> Terminator/1
  MATLAB Function/2(y) -> Terminator1/1
  Zero-Order Hold/1 -> " [x y theta]"/1
  Zero-Order Hold1/1 -> " [x y theta]1"/1
  MATLAB Function3/1(vref) -> Mux6/1
  MATLAB Function3/2(wref) -> Mux6/2
  Subscribe1/1 -> MATLAB Function3/1(IsNew)
  Subscribe1/2 -> MATLAB Function3/2(cmdMsg)
  Mux6/1 -> vw1/1

== system b6_pfc_rl/ROS_simulation/ros6 ==
  x-y-yaw1 : Inport
  do1t : Inport  Port=2
  " [x y theta]" : Demux  Outputs=3
  " [x y theta]1" : Demux  Outputs=3
  Blank Message : robotlib/Blank Message  messageClass=Message  entityType=nav_msgs/Odometry  messageType=nav_msgs/Odometry  SampleTime=inf  legacyBusStruct=off
  Bus Assignment1 : BusAssignment  DialogController=Simulink.DDGSource_BusAssignment  AssignedSignals=Pose.Pose.Position.X,Pose.Pose.Position.Y,Pose.Pose.Orientation.Z,Pose.Pose.Orientation.W,Twist.Twist.Linear.X,Twist.Twist.Linear.Y,Twist.Twist.Angular.Z
  MATLAB Function : MATLAB Function  TreatAsAtomicUnit=on
  MATLAB Function3 : MATLAB Function  TreatAsAtomicUnit=on
  Mux6 : Mux  Inputs=2
  Publish2 : robotlib/Publish  topicSource=Specify your own  topic=/robot_6/pose  messageType=nav_msgs/Odometry  legacyBusStruct=off  messageQueueLength=105
  Subscribe1 : robotlib/Subscribe  topicSource=Specify your own  topic=/robot_6/cmd_vel  messageType=geometry_msgs/Twist  SampleTime=-1  legacyBusStruct=off  messageQueueLength=51
  Terminator : Terminator
  Terminator1 : Terminator
  Zero-Order Hold : ZeroOrderHold  SampleTime=0.1
  Zero-Order Hold1 : ZeroOrderHold  SampleTime=0.1
  vw1 : Outport
  wires:
  " [x y theta]"/1 -> Bus Assignment1/2
  Blank Message/1 -> Bus Assignment1/1
  x-y-yaw1/1 -> Zero-Order Hold/1
  " [x y theta]"/2 -> Bus Assignment1/3
  " [x y theta]1"/2 -> Bus Assignment1/7
  " [x y theta]"/3 -> MATLAB Function/1(yaw)
  " [x y theta]1"/3 -> Bus Assignment1/8
  MATLAB Function/4(w) -> Bus Assignment1/5
  MATLAB Function/3(z) -> Bus Assignment1/4
  " [x y theta]1"/1 -> Bus Assignment1/6
  Bus Assignment1/1 -> Publish2/1
  do1t/1 -> Zero-Order Hold1/1
  MATLAB Function/1(x) -> Terminator/1
  MATLAB Function/2(y) -> Terminator1/1
  MATLAB Function3/1(vref) -> Mux6/1
  MATLAB Function3/2(wref) -> Mux6/2
  Subscribe1/1 -> MATLAB Function3/1(IsNew)
  Subscribe1/2 -> MATLAB Function3/2(cmdMsg)
  Mux6/1 -> vw1/1
  Zero-Order Hold/1 -> " [x y theta]"/1
  Zero-Order Hold1/1 -> " [x y theta]1"/1

== system b6_pfc_rl/Subsystem/Car Pose Listener ==
  Subscribe : robotlib/Subscribe  topicSource=Specify your own  topic=/robot_1/pose  messageType=nav_msgs/Odometry  SampleTime=-1  legacyBusStruct=off  messageQueueLength=51
  Subscribe1 : robotlib/Subscribe  topicSource=Specify your own  topic=/robot_1/odometry  messageType=geometry_msgs/Twist  SampleTime=-1  legacyBusStruct=off  messageQueueLength=51
  Subsystem : Subsystem
  pose x-y-yaw : Outport
  wires:
  Subscribe/1 -> Subsystem/1(poseNew)  "IsNew"
  Subscribe/2 -> Subsystem/2(poseMsg)
  Subscribe1/1 -> Subsystem/3(VW_New)  "IsNew"
  Subscribe1/2 -> Subsystem/4(VW_Msg)
  Subsystem/1(pose) -> pose x-y-yaw/1

== system b6_pfc_rl/Subsystem/Car Pose Listener1 ==
  Subscribe : robotlib/Subscribe  topicSource=Specify your own  topic=/robot_2/pose  messageType=nav_msgs/Odometry  SampleTime=-1  legacyBusStruct=off  messageQueueLength=51
  Subscribe1 : robotlib/Subscribe  topicSource=Specify your own  topic=/robot_2/odometry  messageType=geometry_msgs/Twist  SampleTime=-1  legacyBusStruct=off  messageQueueLength=51
  Subsystem : Subsystem
  pose x-y-yaw : Outport
  wires:
  Subscribe/1 -> Subsystem/1(poseNew)  "IsNew"
  Subscribe/2 -> Subsystem/2(poseMsg)
  Subscribe1/2 -> Subsystem/4(VW_Msg)
  Subscribe1/1 -> Subsystem/3(VW_New)  "IsNew"
  Subsystem/1(pose) -> pose x-y-yaw/1

== system b6_pfc_rl/Subsystem/Car Pose Listener2 ==
  Subscribe : robotlib/Subscribe  topicSource=Specify your own  topic=/robot_3/pose  messageType=nav_msgs/Odometry  SampleTime=-1  legacyBusStruct=off  messageQueueLength=51
  Subscribe1 : robotlib/Subscribe  topicSource=Specify your own  topic=/robot_3/odometry  messageType=geometry_msgs/Twist  SampleTime=-1  legacyBusStruct=off  messageQueueLength=51
  Subsystem : Subsystem
  pose x-y-yaw : Outport
  wires:
  Subscribe/1 -> Subsystem/1(poseNew)  "IsNew"
  Subscribe/2 -> Subsystem/2(poseMsg)
  Subscribe1/1 -> Subsystem/3(VW_New)  "IsNew"
  Subscribe1/2 -> Subsystem/4(VW_Msg)
  Subsystem/1(pose) -> pose x-y-yaw/1

== system b6_pfc_rl/Subsystem/Car Pose Listener3 ==
  Subscribe : robotlib/Subscribe  topicSource=Specify your own  topic=/robot_4/pose  messageType=nav_msgs/Odometry  SampleTime=-1  legacyBusStruct=off  messageQueueLength=51
  Subscribe1 : robotlib/Subscribe  topicSource=Specify your own  topic=/robot_4/odometry  messageType=geometry_msgs/Twist  SampleTime=-1  legacyBusStruct=off  messageQueueLength=51
  Subsystem : Subsystem
  pose x-y-yaw : Outport
  wires:
  Subscribe/1 -> Subsystem/1(poseNew)  "IsNew"
  Subscribe/2 -> Subsystem/2(poseMsg)
  Subscribe1/1 -> Subsystem/3(VW_New)  "IsNew"
  Subscribe1/2 -> Subsystem/4(VW_Msg)
  Subsystem/1(pose) -> pose x-y-yaw/1

== system b6_pfc_rl/Subsystem/Car Pose Listener4 ==
  Subscribe : robotlib/Subscribe  topicSource=Specify your own  topic=/robot_5/pose  messageType=nav_msgs/Odometry  SampleTime=-1  legacyBusStruct=off  messageQueueLength=51
  Subscribe1 : robotlib/Subscribe  topicSource=Specify your own  topic=/robot_5/odometry  messageType=geometry_msgs/Twist  SampleTime=-1  legacyBusStruct=off  messageQueueLength=51
  Subsystem : Subsystem
  pose x-y-yaw : Outport
  wires:
  Subscribe/1 -> Subsystem/1(poseNew)  "IsNew"
  Subscribe/2 -> Subsystem/2(poseMsg)
  Subscribe1/1 -> Subsystem/3(VW_New)  "IsNew"
  Subscribe1/2 -> Subsystem/4(VW_Msg)
  Subsystem/1(pose) -> pose x-y-yaw/1

== system b6_pfc_rl/Subsystem/Car Pose Listener5 ==
  Subscribe : robotlib/Subscribe  topicSource=Specify your own  topic=/robot_6/pose  messageType=nav_msgs/Odometry  SampleTime=-1  legacyBusStruct=off  messageQueueLength=51
  Subscribe1 : robotlib/Subscribe  topicSource=Specify your own  topic=/robot_6/odometry  messageType=geometry_msgs/Twist  SampleTime=-1  legacyBusStruct=off  messageQueueLength=51
  Subsystem : Subsystem
  pose x-y-yaw : Outport
  wires:
  Subscribe/1 -> Subsystem/1(poseNew)  "IsNew"
  Subscribe/2 -> Subsystem/2(poseMsg)
  Subscribe1/1 -> Subsystem/3(VW_New)  "IsNew"
  Subscribe1/2 -> Subsystem/4(VW_Msg)
  Subsystem/1(pose) -> pose x-y-yaw/1

== system b6_pfc_rl/Subsystem/Command Velocity Publisher ==
  v : Inport
  w : Inport  Port=2
  Blank Message : robotlib/Blank Message  messageClass=Message  entityType=geometry_msgs/Twist  messageType=geometry_msgs/Twist  SampleTime=inf  legacyBusStruct=off
  Bus Assignment1 : BusAssignment  DialogController=Simulink.DDGSource_BusAssignment  AssignedSignals=Linear.X,Angular.Z
  Publish2 : robotlib/Publish  topicSource=Specify your own  topic=/robot_1/cmd_vel  messageType=geometry_msgs/Twist  legacyBusStruct=off  messageQueueLength=105
  wires:
  Bus Assignment1/1 -> Publish2/1
  Blank Message/1 -> Bus Assignment1/1
  v/1 -> Bus Assignment1/2
  w/1 -> Bus Assignment1/3

== system b6_pfc_rl/Subsystem/Command Velocity Publisher1 ==
  v : Inport
  w : Inport  Port=2
  Blank Message : robotlib/Blank Message  messageClass=Message  entityType=geometry_msgs/Twist  messageType=geometry_msgs/Twist  SampleTime=inf  legacyBusStruct=off
  Bus Assignment1 : BusAssignment  DialogController=Simulink.DDGSource_BusAssignment  AssignedSignals=Linear.X,Angular.Z
  Publish2 : robotlib/Publish  topicSource=Specify your own  topic=/robot_2/cmd_vel  messageType=geometry_msgs/Twist  legacyBusStruct=off  messageQueueLength=105
  wires:
  Bus Assignment1/1 -> Publish2/1
  Blank Message/1 -> Bus Assignment1/1
  v/1 -> Bus Assignment1/2
  w/1 -> Bus Assignment1/3

== system b6_pfc_rl/Subsystem/Command Velocity Publisher2 ==
  v : Inport
  w : Inport  Port=2
  Blank Message : robotlib/Blank Message  messageClass=Message  entityType=geometry_msgs/Twist  messageType=geometry_msgs/Twist  SampleTime=inf  legacyBusStruct=off
  Bus Assignment1 : BusAssignment  DialogController=Simulink.DDGSource_BusAssignment  AssignedSignals=Linear.X,Angular.Z
  Publish2 : robotlib/Publish  topicSource=Specify your own  topic=/robot_3/cmd_vel  messageType=geometry_msgs/Twist  legacyBusStruct=off  messageQueueLength=105
  wires:
  Bus Assignment1/1 -> Publish2/1
  Blank Message/1 -> Bus Assignment1/1
  v/1 -> Bus Assignment1/2
  w/1 -> Bus Assignment1/3

== system b6_pfc_rl/Subsystem/Command Velocity Publisher3 ==
  v : Inport
  w : Inport  Port=2
  Blank Message : robotlib/Blank Message  messageClass=Message  entityType=geometry_msgs/Twist  messageType=geometry_msgs/Twist  SampleTime=inf  legacyBusStruct=off
  Bus Assignment1 : BusAssignment  DialogController=Simulink.DDGSource_BusAssignment  AssignedSignals=Linear.X,Angular.Z
  Publish2 : robotlib/Publish  topicSource=Specify your own  topic=/robot_4/cmd_vel  messageType=geometry_msgs/Twist  legacyBusStruct=off  messageQueueLength=105
  wires:
  Bus Assignment1/1 -> Publish2/1
  Blank Message/1 -> Bus Assignment1/1
  v/1 -> Bus Assignment1/2
  w/1 -> Bus Assignment1/3

== system b6_pfc_rl/Subsystem/Command Velocity Publisher4 ==
  v : Inport
  w : Inport  Port=2
  Blank Message : robotlib/Blank Message  messageClass=Message  entityType=geometry_msgs/Twist  messageType=geometry_msgs/Twist  SampleTime=inf  legacyBusStruct=off
  Bus Assignment1 : BusAssignment  DialogController=Simulink.DDGSource_BusAssignment  AssignedSignals=Linear.X,Angular.Z
  Publish2 : robotlib/Publish  topicSource=Specify your own  topic=/robot_5/cmd_vel  messageType=geometry_msgs/Twist  legacyBusStruct=off  messageQueueLength=105
  wires:
  Bus Assignment1/1 -> Publish2/1
  Blank Message/1 -> Bus Assignment1/1
  v/1 -> Bus Assignment1/2
  w/1 -> Bus Assignment1/3

== system b6_pfc_rl/Subsystem/Command Velocity Publisher5 ==
  v : Inport
  w : Inport  Port=2
  Blank Message : robotlib/Blank Message  messageClass=Message  entityType=geometry_msgs/Twist  messageType=geometry_msgs/Twist  SampleTime=inf  legacyBusStruct=off
  Bus Assignment1 : BusAssignment  DialogController=Simulink.DDGSource_BusAssignment  AssignedSignals=Linear.X,Angular.Z
  Publish2 : robotlib/Publish  topicSource=Specify your own  topic=/robot_6/cmd_vel  messageType=geometry_msgs/Twist  legacyBusStruct=off  messageQueueLength=105
  wires:
  Bus Assignment1/1 -> Publish2/1
  Blank Message/1 -> Bus Assignment1/1
  v/1 -> Bus Assignment1/2
  w/1 -> Bus Assignment1/3

== system b6_pfc_rl/Subsystem1/car_model1 ==
  note: tr=0.6
      | 4T=0.6
      | 一阶系统的动态性能指标为：td=0.69T，tr=2.20T，ts=3T
  vw1 : Inport
  Demux : Demux  Outputs=2
  Differential Drive Kinematic Model1 : robotmobilelib/Differential Drive Kinematic Model  VehicleInputs=Vehicle Speed & Heading Angular Velocity  WheelRadius=wheelRadius  WheelSpeedRange=[-inf inf]  TrackWidth=robotRadius  InitialState=init_pose_1  SimulateUsing=Interpreted execution
      settings: SourceProductBaseCode=RO
  Simulink顺时针为正 小车逆时针为正 : Gain  Gain=ks
  Transfer Fcn : TransferFcn  Denominator=[0.15 1]
  Transfer Fcn1 : TransferFcn  Denominator=[0.16 1]
  x-y-yaw : Outport
  dot : Outport  Port=2
  wires:
  Simulink顺时针为正 小车逆时针为正/1 -> Transfer Fcn1/1
  Transfer Fcn/1 -> Differential Drive Kinematic Model1/1
  Demux/1 -> Transfer Fcn/1
  Transfer Fcn1/1 -> Differential Drive Kinematic Model1/2
  Demux/2 -> Simulink顺时针为正 小车逆时针为正/1
  vw1/1 -> Demux/1
  Differential Drive Kinematic Model1/1 -> x-y-yaw/1
  Differential Drive Kinematic Model1/2 -> dot/1

== system b6_pfc_rl/Subsystem1/car_model2 ==
  note: tr=0.6
      | 4T=0.6
      | 一阶系统的动态性能指标为：td=0.69T，tr=2.20T，ts=3T
  vw1 : Inport
  Demux : Demux  Outputs=2
  Differential Drive Kinematic Model1 : robotmobilelib/Differential Drive Kinematic Model  VehicleInputs=Vehicle Speed & Heading Angular Velocity  WheelRadius=wheelRadius  WheelSpeedRange=[-inf inf]  TrackWidth=robotRadius  InitialState=init_pose_2  SimulateUsing=Interpreted execution
      settings: SourceProductBaseCode=RO
  Simulink顺时针为正 小车逆时针为正 : Gain  Gain=ks
  Transfer Fcn : TransferFcn  Denominator=[0.15 1]
  Transfer Fcn1 : TransferFcn  Denominator=[0.16 1]
  x-y-yaw : Outport
  dot : Outport  Port=2
  wires:
  Simulink顺时针为正 小车逆时针为正/1 -> Transfer Fcn1/1
  Transfer Fcn/1 -> Differential Drive Kinematic Model1/1
  Demux/1 -> Transfer Fcn/1
  Transfer Fcn1/1 -> Differential Drive Kinematic Model1/2
  Demux/2 -> Simulink顺时针为正 小车逆时针为正/1
  vw1/1 -> Demux/1
  Differential Drive Kinematic Model1/1 -> x-y-yaw/1
  Differential Drive Kinematic Model1/2 -> dot/1

== system b6_pfc_rl/Subsystem1/car_model3 ==
  note: tr=0.6
      | 4T=0.6
      | 一阶系统的动态性能指标为：td=0.69T，tr=2.20T，ts=3T
  vw1 : Inport
  Demux : Demux  Outputs=2
  Differential Drive Kinematic Model1 : robotmobilelib/Differential Drive Kinematic Model  VehicleInputs=Vehicle Speed & Heading Angular Velocity  WheelRadius=wheelRadius  WheelSpeedRange=[-inf inf]  TrackWidth=robotRadius  InitialState=init_pose_3  SimulateUsing=Interpreted execution
      settings: SourceProductBaseCode=RO
  Simulink顺时针为正 小车逆时针为正 : Gain  Gain=ks
  Transfer Fcn : TransferFcn  Denominator=[0.15 1]
  Transfer Fcn1 : TransferFcn  Denominator=[0.16 1]
  x-y-yaw : Outport
  dot : Outport  Port=2
  wires:
  Simulink顺时针为正 小车逆时针为正/1 -> Transfer Fcn1/1
  Transfer Fcn/1 -> Differential Drive Kinematic Model1/1
  Demux/1 -> Transfer Fcn/1
  Transfer Fcn1/1 -> Differential Drive Kinematic Model1/2
  Demux/2 -> Simulink顺时针为正 小车逆时针为正/1
  vw1/1 -> Demux/1
  Differential Drive Kinematic Model1/1 -> x-y-yaw/1
  Differential Drive Kinematic Model1/2 -> dot/1

== system b6_pfc_rl/Subsystem1/car_model4 ==
  note: tr=0.6
      | 4T=0.6
      | 一阶系统的动态性能指标为：td=0.69T，tr=2.20T，ts=3T
  vw1 : Inport
  Demux : Demux  Outputs=2
  Differential Drive Kinematic Model1 : robotmobilelib/Differential Drive Kinematic Model  VehicleInputs=Vehicle Speed & Heading Angular Velocity  WheelRadius=wheelRadius  WheelSpeedRange=[-inf inf]  TrackWidth=robotRadius  InitialState=init_pose_4  SimulateUsing=Interpreted execution
      settings: SourceProductBaseCode=RO
  Simulink顺时针为正 小车逆时针为正 : Gain  Gain=ks
  Transfer Fcn : TransferFcn  Denominator=[0.15 1]
  Transfer Fcn1 : TransferFcn  Denominator=[0.16 1]
  x-y-yaw : Outport
  dot : Outport  Port=2
  wires:
  Simulink顺时针为正 小车逆时针为正/1 -> Transfer Fcn1/1
  Transfer Fcn/1 -> Differential Drive Kinematic Model1/1
  Demux/1 -> Transfer Fcn/1
  Transfer Fcn1/1 -> Differential Drive Kinematic Model1/2
  Demux/2 -> Simulink顺时针为正 小车逆时针为正/1
  vw1/1 -> Demux/1
  Differential Drive Kinematic Model1/1 -> x-y-yaw/1
  Differential Drive Kinematic Model1/2 -> dot/1

== system b6_pfc_rl/Subsystem1/car_model5 ==
  note: tr=0.6
      | 4T=0.6
      | 一阶系统的动态性能指标为：td=0.69T，tr=2.20T，ts=3T
  vw1 : Inport
  Demux : Demux  Outputs=2
  Differential Drive Kinematic Model1 : robotmobilelib/Differential Drive Kinematic Model  VehicleInputs=Vehicle Speed & Heading Angular Velocity  WheelRadius=wheelRadius  WheelSpeedRange=[-inf inf]  TrackWidth=robotRadius  InitialState=init_pose_5  SimulateUsing=Interpreted execution
      settings: SourceProductBaseCode=RO
  Simulink顺时针为正 小车逆时针为正 : Gain  Gain=ks
  Transfer Fcn : TransferFcn  Denominator=[0.15 1]
  Transfer Fcn1 : TransferFcn  Denominator=[0.16 1]
  x-y-yaw : Outport
  dot : Outport  Port=2
  wires:
  Simulink顺时针为正 小车逆时针为正/1 -> Transfer Fcn1/1
  Transfer Fcn/1 -> Differential Drive Kinematic Model1/1
  Demux/1 -> Transfer Fcn/1
  Transfer Fcn1/1 -> Differential Drive Kinematic Model1/2
  Demux/2 -> Simulink顺时针为正 小车逆时针为正/1
  vw1/1 -> Demux/1
  Differential Drive Kinematic Model1/1 -> x-y-yaw/1
  Differential Drive Kinematic Model1/2 -> dot/1

== system b6_pfc_rl/Subsystem1/car_model6 ==
  note: tr=0.6
      | 4T=0.6
      | 一阶系统的动态性能指标为：td=0.69T，tr=2.20T，ts=3T
  vw1 : Inport
  Demux : Demux  Outputs=2
  Differential Drive Kinematic Model1 : robotmobilelib/Differential Drive Kinematic Model  VehicleInputs=Vehicle Speed & Heading Angular Velocity  WheelRadius=wheelRadius  WheelSpeedRange=[-inf inf]  TrackWidth=robotRadius  InitialState=init_pose_6  SimulateUsing=Interpreted execution
      settings: SourceProductBaseCode=RO
  Simulink顺时针为正 小车逆时针为正 : Gain  Gain=ks
  Transfer Fcn : TransferFcn  Denominator=[0.15 1]
  Transfer Fcn1 : TransferFcn  Denominator=[0.16 1]
  x-y-yaw : Outport
  dot : Outport  Port=2
  wires:
  Simulink顺时针为正 小车逆时针为正/1 -> Transfer Fcn1/1
  Transfer Fcn/1 -> Differential Drive Kinematic Model1/1
  Demux/1 -> Transfer Fcn/1
  Transfer Fcn1/1 -> Differential Drive Kinematic Model1/2
  Demux/2 -> Simulink顺时针为正 小车逆时针为正/1
  vw1/1 -> Demux/1
  Differential Drive Kinematic Model1/1 -> x-y-yaw/1
  Differential Drive Kinematic Model1/2 -> dot/1

== system b6_pfc_rl/controller/Ego Car 1 ==
  pose1 : Inport
  pose2 : Inport  Port=2
  leader_linear_vel : Inport  Port=3
  ego_linear_vel : Inport  Port=4
  ego_omega_vel : Inport  Port=5
  Delay : Delay  DelayLength=1  InitialCondition=0
  Signal Process : MATLAB Function  TreatAsAtomicUnit=on
  obs : Outport
  obs_flag : Outport  Port=2
  wires:
  pose1/1 -> Signal Process/1(pose1)
  Signal Process/1(observation) -> obs/1
  leader_linear_vel/1 -> Signal Process/3(leader_linear_vel)
  ego_omega_vel/1 -> Signal Process/5(ego_omega_vel), Delay/1
  pose2/1 -> Signal Process/2(pose2)
  ego_linear_vel/1 -> Signal Process/4(ego_linear_vel)
  Signal Process/2(obs_flag) -> obs_flag/1
  Delay/1 -> Signal Process/6(last_ego_omega_vel)

== system b6_pfc_rl/controller/Ego Car 2 ==
  pose1 : Inport
  pose2 : Inport  Port=2
  leader_linear_vel : Inport  Port=3
  ego_linear_vel : Inport  Port=4
  ego_omega_vel : Inport  Port=5
  Delay : Delay  DelayLength=1  InitialCondition=0
  Signal Process : MATLAB Function  TreatAsAtomicUnit=on
  obs : Outport
  obs_flag : Outport  Port=2
  wires:
  pose1/1 -> Signal Process/1(pose1)
  Signal Process/1(observation) -> obs/1
  leader_linear_vel/1 -> Signal Process/3(leader_linear_vel)
  ego_omega_vel/1 -> Signal Process/5(ego_omega_vel), Delay/1
  pose2/1 -> Signal Process/2(pose2)
  ego_linear_vel/1 -> Signal Process/4(ego_linear_vel)
  Signal Process/2(obs_flag) -> obs_flag/1
  Delay/1 -> Signal Process/6(last_ego_omega_vel)

== system b6_pfc_rl/controller/Ego Car 3 ==
  pose1 : Inport
  pose2 : Inport  Port=2
  leader_linear_vel : Inport  Port=3
  ego_linear_vel : Inport  Port=4
  ego_omega_vel : Inport  Port=5
  Delay : Delay  DelayLength=1  InitialCondition=0
  Signal Process : MATLAB Function  TreatAsAtomicUnit=on
  obs : Outport
  obs_flag : Outport  Port=2
  wires:
  pose1/1 -> Signal Process/1(pose1)
  Signal Process/1(observation) -> obs/1
  leader_linear_vel/1 -> Signal Process/3(leader_linear_vel)
  ego_omega_vel/1 -> Signal Process/5(ego_omega_vel), Delay/1
  pose2/1 -> Signal Process/2(pose2)
  ego_linear_vel/1 -> Signal Process/4(ego_linear_vel)
  Signal Process/2(obs_flag) -> obs_flag/1
  Delay/1 -> Signal Process/6(last_ego_omega_vel)
